simulink model "Torque_Vectoring"  (R2020a)
settings: Solver=FixedStepDiscrete  StartTime=0.0  StopTime=inf  FixedStep=0.01  RelTol=1e-3  EnableMultiTasking=on
undefined symbols (not defined in the file): T_t, VEH, w_eff_bp
libraries: simulink x4
settings Model: DataDictionary=System_Data_Dictionary.sldd  OrderedModelArguments=off  Creator=koshiro  LastModifiedBy=jchu
settings SolverCC: AutoInsertRateTranBlk=on
settings DataIOCC: ReturnWorkspaceOutputs=off
settings OptimizationCC: UseDivisionForNetSlopeComputation=on
settings DebuggingCC: ArithmeticOperatorsInVariantConditions=warning
settings ModelReferenceCC: ModelReferenceNumInstancesAllowed=Single
settings SFSimCC: CustomCodeUndefinedFunction=UseInterfaceOnly

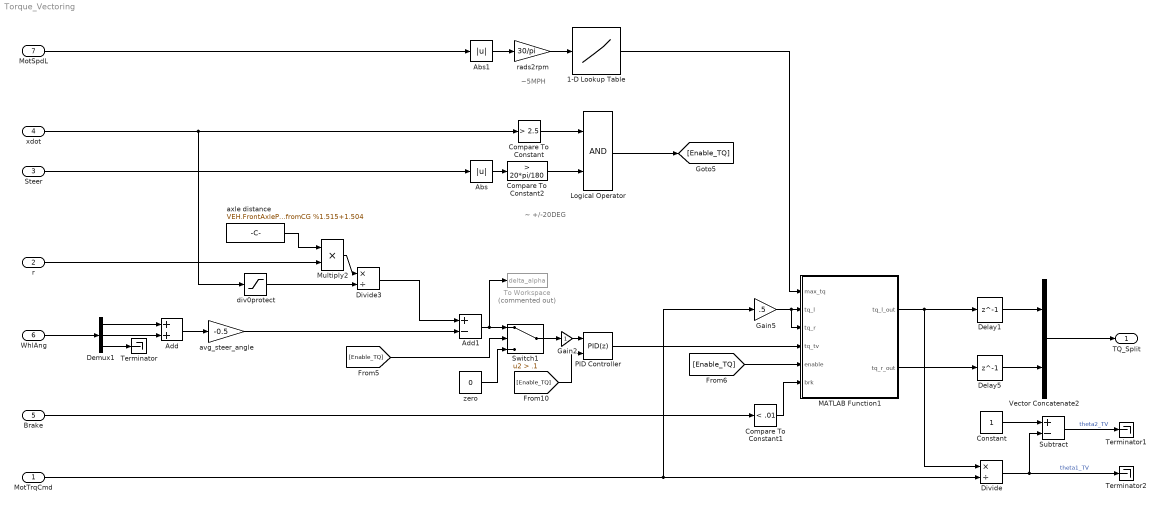
== system Torque_Vectoring ==
  note: ~ +/-20DEG
  note: ~5MPH
  MotTrqCmd : Inport
  r : Inport  Port=2
  Steer : Inport  Port=3
  xdot : Inport  Port=4
  Brake : Inport  Port=5
  WhlAng : Inport  Port=6
  MotSpdL : Inport  Port=7
  1-D Lookup Table : Lookup_n-D  NumberOfTableDimensions=1  BreakpointsForDimension1=w_eff_bp  Table=T_t  ExtrapMethod=Clip  UseLastTableValue=on  InternalRulePriority=Speed  RndMeth=Simplest  InputSameDT=on
  Abs : Abs
  Abs1 : Abs
  Add : Sum
  Add1 : Sum  Inputs=+-
  Compare To Constant : simulink/Logic and Bit Operations/Compare To Constant  relop=>  const=2.5  OutDataTypeStr=boolean
  Compare To Constant1 : simulink/Logic and Bit Operations/Compare To Constant  relop=<  const=.01  OutDataTypeStr=boolean
  Compare To Constant2 : simulink/Logic and Bit Operations/Compare To Constant  relop=>  const=20*pi/180  OutDataTypeStr=boolean
  Constant : Constant
  Delay1 : Delay  DelayLength=1  InitialCondition=0
  Delay5 : Delay  DelayLength=1  InitialCondition=0
  Demux1 : Demux  Outputs=[1 1 2]
  Divide : Product  Inputs=*/
  Divide3 : Product  Inputs=*/
  Gain2 : Gain
  Gain5 : Gain  Gain=.5
  Logical Operator : Logic  AllPortsSameDT=off  OutDataTypeStr=boolean
  MATLAB Function1 : MATLAB Function  TreatAsAtomicUnit=on
  Multiply2 : Product
  PID Controller : simulink/Continuous/PID Controller  Controller=PID  Form=Parallel  TimeDomain=Discrete-time  UseExternalTs=off  SampleTime=-1  IntegratorMethod=Forward Euler  FilterMethod=Forward Euler  ControllerParametersSource=internal  P=-1000*2  I=-100*5  D=0  UseFilter=on  N=1  TunerSelectOption=Transfer Function Based (PID Tuner App)  InitialConditionSource=internal  InitialConditionForIntegrator=0  InitialConditionForFilter=0  DifferentiatorICPrevScaledInput=0  ExternalReset=either  TrackingMode=off  Kt=1  LimitOutput=off  UpperSaturationLimit=inf  LowerSaturationLimit=-inf  LinearizeAsGain=on  AntiWindupMode=none  Kb=1  POutMin=[]  POutMax=[]  IOutMin=[]  IOutMax=[]  DOutMin=[]  DOutMax=[]  NOutMin=[]  NOutMax=[]  SumOutMin=[]  SumOutMax=[]  SaturationOutMin=[]  SaturationOutMax=[]  PParamMin=[]  PParamMax=[]  IParamMin=[]  IParamMax=[]  DParamMin=[]  DParamMax=[]  NParamMin=[]  NParamMax=[]  KbParamMin=[]  KbParamMax=[]  KtParamMin=[]  KtParamMax=[]  KbOutMin=[]  KbOutMax=[]  KtOutMin=[]  KtOutMax=[]  IntegratorOutMin=[]  IntegratorOutMax=[]  FilterOutMin=[]  FilterOutMax=[]  SumI1OutMin=[]  SumI1OutMax=[]  SumI2OutMin=[]  SumI2OutMax=[]  SumI3OutMin=[]  SumI3OutMax=[]  SumI4OutMin=[]  SumI4OutMax=[]  SumDOutMin=[]  SumDOutMax=[]  DifferentiatorOutMin=[]  DifferentiatorOutMax=[]  FilterDiffOutCoefMin=[]  FilterDiffOutCoefMax=[]  ReciprocalOutMin=[]  ReciprocalOutMax=[]  SumDenOutMin=[]  SumDenOutMax=[]  SumNumOutMin=[]  SumNumOutMax=[]  DivideOutMin=[]  DivideOutMax=[]  UdiffTsProdOutMin=[]  UdiffTsProdOutMax=[]  NTsProdOutMin=[]  NTsProdOutMax=[]  UintegralTsProdOutMin=[]  UintegralTsProdOutMax=[]  UngainTsProdOutMin=[]  UngainTsProdOutMax=[]  IntegratorContinuousStateAttributes=''  IntegratorStateMustResolveToSignalObject=off  IntegratorRTWStateStorageClass=Auto  FilterContinuousStateAttributes=''  FilterStateMustResolveToSignalObject=off  FilterRTWStateStorageClass=Auto  ParallelPVariant=InternalParameters  IdealPVariant=Disabled  IVariant=InternalParameters  DVariant=InternalParameters  IntegratorVariant=Discrete  SatVariant=Disabled  AWVariant=Passthrough  PCopyVariant=Disabled  TRVariant=Disabled  FdbkBlocksVariant=Forward  IdealPFdbkVariant=Disabled  SatFdbkVariant=Disabled  DerivativeFilterVariant=ForwardEulerFilter  NVariant=InternalParameters  NCopyVariant=Disabled  FilterICVariant=InternalICsFilter  IntegratorICVariant=InternalICs  ExternalResetVariant=ExternalReset  TRSumVariant=Passthrough  SumFdbkVariant=Disabled  SumVariant=Sum_PID  TsampFilterVariant=InternalTs  TsampNgainVariant=Passthrough  TsampIntegralVariant=Passthrough
  Subtract : Sum  Inputs=+-
  Switch1 : Switch  Criteria=u2 > Threshold  Threshold=.1
  Terminator : Terminator
  Terminator1 : Terminator
  Terminator2 : Terminator
  To Workspace : ToWorkspace  Commented=on  VariableName=delta_alpha  SaveFormat=Timeseries  SampleTime=-1
  Vector Concatenate2 : Concatenate
  avg_steer_angle : Gain  Gain=-0.5
  axle distance : Constant  Value=VEH.FrontAxlePositionfromCG + VEH.RearAxlePositionfromCG %1.515+1.504
  div0protect : Saturate  UpperLimit=inf  LowerLimit=0.01  ZeroCross=off
  rads2rpm : Gain  Gain=30/pi
  zero : Constant  Value=0
  TQ_Split : Outport  VectorParamsAs1DForOutWhenUnconnected=off
  wires:
  MotSpdL/1 -> Abs1/1
  [Enable_TQ] -> PID Controller/2
  MATLAB Function1/1(tq_l_out) -> Delay1/1, Divide/1
  Divide/1 -> Terminator2/1, Subtract/2  "theta1_TV"
  Vector Concatenate2/1 -> TQ_Split/1
  WhlAng/1 -> Demux1/1
  Compare To Constant/1 -> Logical Operator/1
  Delay5/1 -> Vector Concatenate2/2
  Add/1 -> avg_steer_angle/1
  Demux1/3 -> Terminator/1
  Add1/1 -> To Workspace/1, Switch1/1
  MATLAB Function1/2(tq_r_out) -> Delay5/1
  [Enable_TQ] -> Switch1/2
  rads2rpm/1 -> 1-D Lookup Table/1
  Steer/1 -> Abs/1
  Demux1/1 -> Add/1
  Abs/1 -> Compare To Constant2/1
  Delay1/1 -> Vector Concatenate2/1
  zero/1 -> Switch1/3
  [Enable_TQ] -> MATLAB Function1/5(enable)
  Abs1/1 -> rads2rpm/1
  Switch1/1 -> Gain2/1
  Compare To Constant2/1 -> Logical Operator/2
  Compare To Constant1/1 -> MATLAB Function1/6(brk)
  PID Controller/1 -> MATLAB Function1/4(tq_tv)
  Gain2/1 -> PID Controller/1
  axle distance/1 -> Multiply2/1
  avg_steer_angle/1 -> Add1/2
  Constant/1 -> Subtract/1
  xdot/1 -> Compare To Constant/1, div0protect/1
  Divide3/1 -> Add1/1
  1-D Lookup Table/1 -> MATLAB Function1/1(max_tq)
  r/1 -> Multiply2/2
  Multiply2/1 -> Divide3/1
  Demux1/2 -> Add/2
  Brake/1 -> Compare To Constant1/1
  MotTrqCmd/1 -> Divide/2, Gain5/1
  Gain5/1 -> MATLAB Function1/3(tq_r), MATLAB Function1/2(tq_l)
  Logical Operator/1 -> [Enable_TQ]
  Subtract/1 -> Terminator1/1  "theta2_TV"
  div0protect/1 -> Divide3/2

== matlab function Torque_Vectoring/MATLAB Function1 ==
  data: max_tq input; tq_l_out output; tq_l input; tq_r input; tq_r_out output; tq_tv input; enable input; brk input
function [tq_l_out,tq_r_out] = fcn(max_tq,tq_l,tq_r,tq_tv,enable,brk)
% enable:= flag to turn on TV, true if steering wheel is turned and non-zero vehicle speed
% brk:= flag to turn on TV, true if not braking
t_lim=min(max_tq-abs(tq_l),max_tq-abs(tq_r));
delta_t=min(100,min(t_lim,abs(tq_tv)))*sign(tq_tv)*enable;% limit difference in torque between tires to +/-50Nm and to max/min motor torque
if brk>0 % Not braking. Use Torque vectoring
    tq_l_out=(tq_l+delta_t);
    tq_r_out=(tq_r-delta_t);
else % ignore TV
    tq_l_out=tq_l;
    tq_r_out=tq_r;
end
